simulink model "sampleModel1967"  (R2023a)
settings: Solver=VariableStepAuto  StartTime=0.0  StopTime=10.0  RelTol=1e-3
libraries: hdlsllib x4
settings Model: Creator=user1  LastModifiedBy=user1

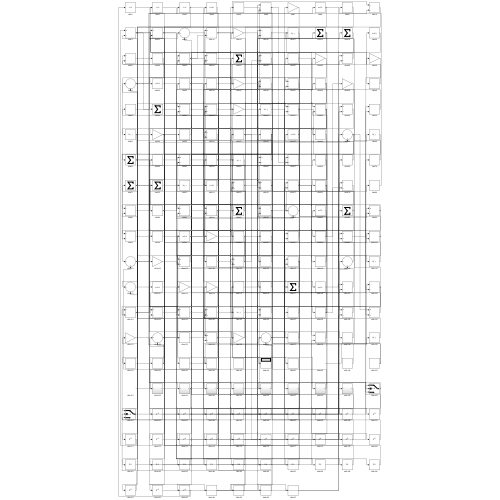
[thumbnail: Simulink's stored preview of the top-level diagram]
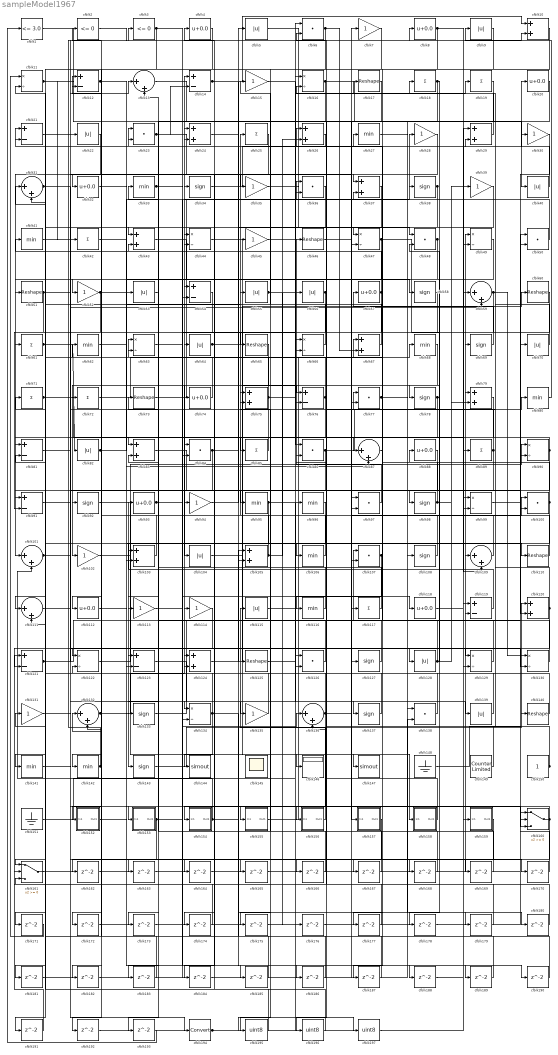
== system sampleModel1967 ==
  cfblk1 : hdlsllib/Logic and Bit Operations/Compare To Constant  relop=<=  const=3.0  OutDataTypeStr=boolean
  cfblk{10,24,26,29,37,43,67,75,79,83,103,105,120,124} (14 alike) : Sum
  cfblk{6,23,36,48,50,77,84,86,97,100,107,126,138} (13 alike) : DotProduct  OutDataTypeStr=Inherit: Inherit via internal rule
  cfblk{13,31,59,87,101,109,111,132,136} (9 alike) : Sum  Inputs=|++
  cfblk{7,15,28,30,35,39,45,52,94,102,113..114,131,135} (14 alike) : Gain
  cfblk{5,9,22,40,53,55..56,64,70,82,104,115,128,139} (14 alike) : Abs  SaturateOnIntegerOverflow=off
  cfblk{27,33,41,62,68,80,95..96,106,116,141..142} (12 alike) : MinMax
  cfblk{34,38,58,69,78,92,98,108,127,133,137,143} (12 alike) : Signum
  cfblk{11,16,44,47,49,63,66,90,99,122,129..130,134} (13 alike) : Product  Inputs=*/  RndMeth=Zero  SaturateOnIntegerOverflow=on
  cfblk{17,46,51,60,65,73,110,125,140} (9 alike) : Reshape
  cfblk{4,8,20,32,57,74,88,93,112,118} (10 alike) : Bias  Bias=0.0  SaturateOnIntegerOverflow=off
  cfblk{18..19,25,42,61,71..72,85,89,117} (10 alike) : Sum  Inputs=+
  cfblk{12,14,21,54,76,81,91,119,121,123} (10 alike) : Sum  Inputs=+-
  cfblk144 : ToWorkspace  VariableName=simout  SaveFormat=Timeseries  SampleTime=-1
  cfblk145 : Scope
      settings: Floating=on
  cfblk146 : Display
  cfblk147 : ToWorkspace  VariableName=simout  SaveFormat=Timeseries  SampleTime=-1
  cfblk148 : Ground
  cfblk149 : hdlsllib/Sources/Counter Limited  uplimit=7  tsamp=-1
  cfblk150 : Constant  SampleTime=-1
  cfblk151 : Ground
  cfblk152 : Subsystem
      settings: LibrarySourceBlock=|
      | hdlsllib/Ports &
      | Subsystems/Subsystem
  cfblk153 : Subsystem
      settings: LibrarySourceBlock=|
      | hdlsllib/Ports &
      | Subsystems/Subsystem
  cfblk154 : Subsystem
      settings: LibrarySourceBlock=|
      | hdlsllib/Ports &
      | Subsystems/Subsystem
  cfblk155 : Subsystem
      settings: LibrarySourceBlock=|
      | hdlsllib/Ports &
      | Subsystems/Subsystem
  cfblk156 : Subsystem
      settings: LibrarySourceBlock=|
      | hdlsllib/Ports &
      | Subsystems/Subsystem
  cfblk157 : Subsystem
      settings: LibrarySourceBlock=|
      | hdlsllib/Ports &
      | Subsystems/Subsystem
  cfblk158 : Subsystem
      settings: LibrarySourceBlock=|
      | hdlsllib/Ports &
      | Subsystems/Subsystem
  cfblk159 : Subsystem
      settings: LibrarySourceBlock=|
      | hdlsllib/Ports &
      | Subsystems/Subsystem
  cfblk160 : Switch  SaturateOnIntegerOverflow=off  InputSameDT=off
  cfblk161 : Switch  SaturateOnIntegerOverflow=off  InputSameDT=off
  cfblk{162..193} (32 alike) : Delay  SampleTime=1
  cfblk194 : DataTypeConversion  SaturateOnIntegerOverflow=off  RndMeth=Floor
  cfblk195 : DataTypeConversion  OutDataTypeStr=uint8  SaturateOnIntegerOverflow=off  RndMeth=Floor
  cfblk196 : DataTypeConversion  OutDataTypeStr=uint8  SaturateOnIntegerOverflow=off  RndMeth=Floor
  cfblk197 : DataTypeConversion  OutDataTypeStr=uint8  SaturateOnIntegerOverflow=off  RndMeth=Floor
  cfblk2 : hdlsllib/Logic and Bit Operations/Compare To Zero  relop=<=  OutDataTypeStr=boolean
  cfblk3 : hdlsllib/Logic and Bit Operations/Compare To Zero  relop=<=  OutDataTypeStr=boolean
  wires:
  cfblk128/1 -> cfblk39/1, cfblk67/1, cfblk48/2
  cfblk135/1 -> cfblk14/1
  cfblk97/1 -> cfblk46/1
  cfblk68/1 -> cfblk102/1
  cfblk142/1 -> cfblk3/1, cfblk2/1
  cfblk84/1 -> cfblk142/1, cfblk128/1
  cfblk47/1 -> cfblk98/1, cfblk84/1
  cfblk61/1 -> cfblk82/1, cfblk134/1
  cfblk34/1 -> cfblk20/1
  cfblk155/1(Out1) -> cfblk68/1
  cfblk80/1 -> cfblk9/1
  cfblk17/1 -> cfblk116/1
  cfblk64/1 -> cfblk147/1, cfblk44/1
  cfblk14/1 -> cfblk10/1, cfblk48/1
  cfblk148/1 -> cfblk120/1
  cfblk122/1 -> cfblk90/1
  cfblk131/1 -> cfblk194/1
  cfblk109/1 -> cfblk88/1
  cfblk50/1 -> cfblk34/1
  cfblk25/1 -> cfblk32/1
  cfblk85/1 -> cfblk83/1
  cfblk160/1 -> cfblk156/1(In1), cfblk163/1
  cfblk5/1 -> cfblk47/1
  cfblk124/1 -> cfblk60/1
  cfblk74/1 -> cfblk63/1
  cfblk30/1 -> cfblk120/2
  cfblk22/1 -> cfblk101/1
  cfblk104/1 -> cfblk146/1
  cfblk44/1 -> cfblk76/1
  cfblk154/1(Out1) -> cfblk101/2, cfblk188/1
  cfblk140/1 -> cfblk49/1
  cfblk73/1 -> cfblk28/1
  cfblk37/1 -> cfblk141/1
  cfblk105/1 -> cfblk23/1, cfblk26/2
  cfblk2/1 -> cfblk10/2
  cfblk156/1(Out1) -> cfblk115/1
  cfblk120/1 -> cfblk121/2, cfblk17/1, cfblk165/1
  cfblk158/1(Out1) -> cfblk6/2
  cfblk69/1 -> cfblk57/1
  cfblk88/1 -> cfblk97/2
  cfblk3/1 -> cfblk66/2, cfblk172/1
  cfblk108/1 -> cfblk25/1
  cfblk33/1 -> cfblk118/1, cfblk85/1
  cfblk72/1 -> cfblk7/1
  cfblk92/1 -> cfblk137/1
  cfblk138/1 -> cfblk114/1
  cfblk45/1 -> cfblk29/2
  cfblk35/1 -> cfblk157/1(In1)
  cfblk133/1 -> cfblk70/1
  cfblk110/1 -> cfblk54/1
  cfblk48/1 -> cfblk112/1, cfblk152/1(In1), cfblk187/1
  cfblk41/1 -> cfblk22/1
  cfblk111/1 -> cfblk155/1(In1)
  cfblk96/1 -> cfblk143/1
  cfblk121/1 -> cfblk107/1, cfblk59/2
  cfblk65/1 -> cfblk104/1
  cfblk149/1 -> cfblk56/1
  cfblk125/1 -> cfblk80/1
  cfblk116/1 -> cfblk63/2
  cfblk20/1 -> cfblk43/1
  cfblk101/1 -> cfblk77/1, cfblk123/1
  cfblk119/1 -> cfblk93/1
  cfblk77/1 -> cfblk108/1, cfblk130/2
  cfblk143/1 -> cfblk140/1
  cfblk4/1 -> cfblk52/1
  cfblk23/1 -> cfblk127/1, cfblk14/2
  cfblk102/1 -> cfblk158/1(In1)
  cfblk67/1 -> cfblk15/1
  cfblk87/1 -> cfblk27/1
  cfblk117/1 -> cfblk24/1
  cfblk126/1 -> cfblk94/1
  cfblk98/1 -> cfblk64/1, cfblk79/2
  cfblk11/1 -> cfblk40/1, cfblk76/2, cfblk42/1
  cfblk49/1 -> cfblk51/1
  cfblk89/1 -> cfblk154/1(In1), cfblk26/1
  cfblk10/1 -> cfblk37/1
  cfblk134/1 -> cfblk144/1, cfblk81/2, cfblk180/1
  cfblk82/1 -> cfblk36/1, cfblk132/2
  cfblk53/1 -> cfblk33/1
  cfblk55/1 -> cfblk18/1, cfblk176/1
  cfblk161/1 -> cfblk109/1
  cfblk137/1 -> cfblk71/1
  cfblk62/1 -> cfblk55/1
  cfblk114/1 -> cfblk122/1
  cfblk153/1(Out1) -> cfblk136/1, cfblk182/1
  cfblk59/1 -> cfblk130/1, cfblk168/1, cfblk195/1
  cfblk16/1 -> cfblk138/1, cfblk193/1
  cfblk1/1 -> cfblk45/1
  cfblk31/1 -> cfblk35/1, cfblk129/1
  cfblk103/1 -> cfblk12/1
  cfblk32/1 -> cfblk54/2
  cfblk123/1 -> cfblk135/1
  cfblk115/1 -> cfblk96/1
  cfblk95/1 -> cfblk139/1, cfblk134/2
  cfblk86/1 -> cfblk69/1, cfblk103/2
  cfblk132/1 -> cfblk124/1, cfblk160/3
  cfblk6/1 -> cfblk61/1, cfblk67/2
  cfblk118/1 -> cfblk89/1
  cfblk43/1 -> cfblk105/2
  cfblk130/1 -> cfblk73/1
  cfblk56/1 -> cfblk92/1, cfblk72/1, cfblk103/1
  cfblk81/1 -> cfblk8/1
  cfblk100/1 -> cfblk21/1, cfblk181/1
  cfblk75/1 -> cfblk19/1, cfblk11/2, cfblk164/1
  cfblk139/1 -> cfblk83/2
  cfblk78/1 -> cfblk177/1, cfblk178/1
  cfblk13/1 -> cfblk117/1
  cfblk26/1 -> cfblk21/2
  cfblk7/1 -> cfblk111/1
  cfblk15/1 -> cfblk86/1
  cfblk127/1 -> cfblk75/1
  cfblk83/1 -> cfblk107/2
  cfblk107/1 -> cfblk166/1, cfblk167/1
  cfblk57/1 -> cfblk133/1, cfblk12/2
  cfblk18/1 -> cfblk78/1, cfblk87/1
  cfblk136/1 -> cfblk119/2, cfblk44/2, cfblk100/1, cfblk174/1
  cfblk66/1 -> cfblk31/2
  cfblk71/1 -> cfblk109/2, cfblk123/2
  cfblk39/1 -> cfblk74/1
  cfblk70/1 -> cfblk37/2
  cfblk106/1 -> cfblk62/1
  cfblk94/1 -> cfblk5/1
  cfblk90/1 -> cfblk111/2, cfblk81/1
  cfblk151/1 -> cfblk16/1
  cfblk141/1 -> cfblk153/1(In1)
  cfblk46/1 -> cfblk160/2
  cfblk19/1 -> cfblk36/2
  cfblk8/1 -> cfblk65/1, cfblk100/2
  cfblk40/1 -> cfblk30/1
  cfblk60/1 -> cfblk161/1
  cfblk29/1 -> cfblk16/2
  cfblk42/1 -> cfblk58/1
  cfblk51/1 -> cfblk99/2, cfblk91/2
  cfblk21/1 -> cfblk13/1
  cfblk99/1 -> cfblk50/2
  cfblk129/1 -> cfblk86/2
  cfblk52/1 -> cfblk87/2, cfblk190/1, cfblk191/1
  cfblk12/1 -> cfblk53/1, cfblk110/1
  cfblk24/1 -> cfblk125/1
  cfblk38/1 -> cfblk106/1, cfblk175/1
  cfblk9/1 -> cfblk91/1
  cfblk93/1 -> cfblk38/1, cfblk95/1
  cfblk150/1 -> cfblk41/1, cfblk79/1
  cfblk76/1 -> cfblk13/2, cfblk113/1
  cfblk36/1 -> cfblk162/1
  cfblk162/1 -> cfblk90/2
  cfblk163/1 -> cfblk29/1
  cfblk164/1 -> cfblk49/2
  cfblk165/1 -> cfblk97/1
  cfblk166/1 -> cfblk43/2
  cfblk167/1 -> cfblk75/2
  cfblk168/1 -> cfblk23/2
  cfblk91/1 -> cfblk169/1
  cfblk169/1 -> cfblk24/2
  cfblk113/1 -> cfblk170/1
  cfblk170/1 -> cfblk160/1
  cfblk79/1 -> cfblk171/1
  cfblk171/1 -> cfblk11/1
  cfblk172/1 -> cfblk126/2
  cfblk157/1(Out1) -> cfblk173/1
  cfblk173/1 -> cfblk47/2
  cfblk174/1 -> cfblk121/1
  cfblk175/1 -> cfblk59/1
  cfblk176/1 -> cfblk50/1
  cfblk177/1 -> cfblk136/2
  cfblk178/1 -> cfblk119/1
  cfblk27/1 -> cfblk179/1
  cfblk179/1 -> cfblk6/1
  cfblk180/1 -> cfblk31/1
  cfblk181/1 -> cfblk138/2
  cfblk182/1 -> cfblk84/2
  cfblk54/1 -> cfblk183/1
  cfblk183/1 -> cfblk122/2
  cfblk28/1 -> cfblk184/1
  cfblk184/1 -> cfblk77/2
  cfblk112/1 -> cfblk185/1
  cfblk185/1 -> cfblk124/2
  cfblk152/1(Out1) -> cfblk186/1
  cfblk186/1 -> cfblk66/1
  cfblk187/1 -> cfblk161/3
  cfblk188/1 -> cfblk129/2
  cfblk63/1 -> cfblk189/1
  cfblk189/1 -> cfblk105/1
  cfblk190/1 -> cfblk132/1
  cfblk191/1 -> cfblk161/2
  cfblk58/1 -> cfblk192/1
  cfblk192/1 -> cfblk99/1
  cfblk193/1 -> cfblk1/1
  cfblk194/1 -> cfblk126/1, cfblk197/1
  cfblk195/1 -> cfblk131/1
  cfblk159/1(Out1) -> cfblk196/1
  cfblk196/1 -> cfblk4/1
  cfblk197/1 -> cfblk159/1(In1)

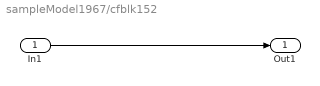
== system sampleModel1967/cfblk152 ==
  In1 : Inport
  Out1 : Outport
  wires:
  In1/1 -> Out1/1

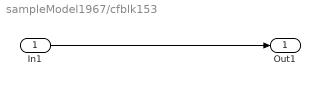
== system sampleModel1967/cfblk153 ==
  In1 : Inport
  Out1 : Outport
  wires:
  In1/1 -> Out1/1

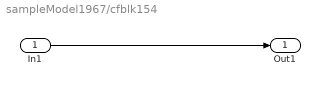
== system sampleModel1967/cfblk154 ==
  In1 : Inport
  Out1 : Outport
  wires:
  In1/1 -> Out1/1

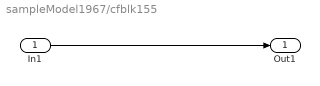
== system sampleModel1967/cfblk155 ==
  In1 : Inport
  Out1 : Outport
  wires:
  In1/1 -> Out1/1

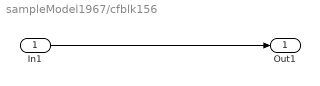
== system sampleModel1967/cfblk156 ==
  In1 : Inport
  Out1 : Outport
  wires:
  In1/1 -> Out1/1

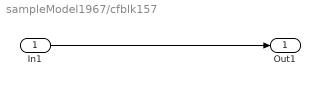
== system sampleModel1967/cfblk157 ==
  In1 : Inport
  Out1 : Outport
  wires:
  In1/1 -> Out1/1

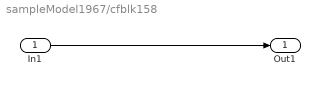
== system sampleModel1967/cfblk158 ==
  In1 : Inport
  Out1 : Outport
  wires:
  In1/1 -> Out1/1

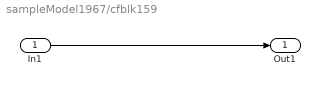
== system sampleModel1967/cfblk159 ==
  In1 : Inport
  Out1 : Outport
  wires:
  In1/1 -> Out1/1
